simulink model "PMSM_FOC_Traction"  (R2020b)
settings: Solver=FixedStepAuto  StartTime=0.0  StopTime=10  RelTol=1e-3
model workspace (MAT data in the model file):
  wc : Simulink.Parameter (value not decoded)
values from neighbouring files (symbols this model uses):
  Cosine_table = 1.0 0.99999529 0.99999058 0.99998587 0.99998116 0.99996704 0.99995291 0.99993885 0.99992472 0.99990118 0.99987763 0.99985409 0.9998306 0.99979764 0.99976468 0.99973178 0.99969882 0.99965644 0.99961412 0.99957174 0.99952942 0.99947762 0.99942589 0.99937415 0.99932235 0.9992612 0.99920005 0.99913889 0.99907768 0.99900717 0.99893659 0.99886602 0.99879545 0.99871546 0.99863547 0.99855554 0.99847555 0.    [Hall_HSMO_FOC_Data.sldd]    (also in Hall_SMO_FOC_Data.sldd)
  Flux = 0.0109    [G474_FOC_HSMO.sldd]    (also in Hall_HSMO_FOC_Data.sldd = 0.00529276
  MTPA_id_table = 0.22889 0.23462678 0.23770036 0.2381243 0.23591207 0.23107713 0.2236329 0.21359272 0.20096992 0.18577772 0.16802935 0.14773798 0.12491672 0.099578641 0.071736768 0.041404068 0.0085934745 -0.026682133 -0.064409919 -0.10457709 -0.14717092 -0.1921787 -0.2395878 -0.28938559 -0.34155953 -0.39609709 -0.45298585 -0.51221335 -0.57376724 -0.63763517 -0.70380485 -0.77226412 -0.84300071 -0.91600245 -0.991257    [Hall_HSMO_FOC_Data.sldd]    (also in Hall_SMO_FOC_Data.sldd)
  MTPA_iq_table = -1.0417 -0.16083497 0.71926296 1.5985928 2.4771533 3.3549435 4.2319627 5.1082091 5.9836826 6.8583813 7.732305 8.6054525 9.4778223 10.349415 11.220228 12.090261 12.959513 13.827983 14.69567 15.562573 16.428694 17.294027 18.158575 19.022335 19.885307 20.747492 21.608887 22.469492 23.329306 24.188328 25.046556 25.903992 26.760633 27.616482 28.471533 29.325788 30.179247 31.031908 31.883772 32.734837 3    [Hall_HSMO_FOC_Data.sldd]    (also in Hall_SMO_FOC_Data.sldd)
  MTPA_Te_Max = 800.0    [Hall_HSMO_FOC_Data.sldd]    (also in Hall_SMO_FOC_Data.sldd)
  MTPA_Te_Min = 0.0    [Hall_HSMO_FOC_Data.sldd]    (also in Hall_SMO_FOC_Data.sldd)
  Sine_table = 0.0 0.0015339879 0.0030679768 0.0046019657 0.0061359555 0.0076698866 0.0092038177 0.010737749 0.012271681 0.013805497 0.015339312 0.016873131 0.018406944 0.019940587 0.021474229 0.023007872 0.024541514 0.026074925 0.027608337 0.029141748 0.03067516 0.032208283 0.033741407 0.035274528 0.036807653 0.038340431 0.039873205 0.04140598 0.042938754 0.04447113 0.046003502 0.047535874 0.049068246 0.0506001    [Hall_HSMO_FOC_Data.sldd]    (also in Hall_SMO_FOC_Data.sldd)
undefined symbols (not defined in the file or in its folder): CL_Param, ctrlParamsPI, DiscIntNeverNeededParam, Flux_weak, FluxObsever, Hall_Parameter, HFI, inverter, Kiv, Kiw, Kpv, Kpw, magnitude, OPL_Param, pmsm, Resolver_Parameter, sigbuilder_block, SMO, SVPWM, Vdc
libraries: powerlib x29, fl_lib x18, simulink x7, nesl_utility x7, pid_lib x5, dspstat3 x4, eeGeneralControl x4, eeDiscretePi x2, powerlib_extras x1, ee_lib x1
(part 4 of 6)

== system PMSM_FOC_Traction/Motor_Control/Motor_Control_Funtion/Angle_Speed_100us/SMO/Delta_theta ==
  Est_theta : Inport
  Ealpha_est : Inport  Port=2
  Ebeta_est : Inport  Port=3
  Add : Sum
  Add1 : Sum
  Divide : Product  Inputs=*/
  Gain : Gain  Gain=-1
  Math Function : Math  Operator=magnitude^2  SaturateOnIntegerOverflow=on
  Math Function1 : Math  Operator=magnitude^2  SaturateOnIntegerOverflow=on
  Product : Product
  Product1 : Product
  Saturation : Saturate  UpperLimit=inf  LowerLimit=4.0
  Sine_Cosine : Subsystem  TreatAsAtomicUnit=on
      settings: RTWSystemCode=Nonreusable function  RTWFcnNameOpts=Use subsystem name
  Sqrt : Sqrt  SaturateOnIntegerOverflow=on
  delta_theta : Outport
  unit : Outport  Port=2
  wires:
  Est_theta/1 -> Sine_Cosine/1(P)
  Ealpha_est/1 -> Math Function/1, Product/2
  Sine_Cosine/1(Sin) -> Product1/1
  Ebeta_est/1 -> Math Function1/1, Product1/2
  Product/1 -> Add/1
  Product1/1 -> Add/2
  Add/1 -> Gain/1
  Math Function/1 -> Add1/1
  Math Function1/1 -> Add1/2
  Add1/1 -> Sqrt/1
  Sqrt/1 -> Saturation/1
  Gain/1 -> Divide/1
  Saturation/1 -> unit/1, Divide/2
  Divide/1 -> delta_theta/1
  Sine_Cosine/2(Cos) -> Product/1

== system PMSM_FOC_Traction/Motor_Control/Motor_Control_Funtion/Angle_Speed_100us/SMO/PLL_PI ==
  in : Inport
  Add : Sum
  Discrete-Time Integrator : DiscreteIntegrator  SampleTime=Ts  ICPrevOutput=DiscIntNeverNeededParam  ICPrevScaledInput=DiscIntNeverNeededParam
  Gain2 : Gain  Gain=kp
  Gain3 : Gain  Gain=ki
  Saturation : Saturate  UpperLimit=inf  LowerLimit=-inf
  Scope : Scope  NumInputPorts=3
  Out : Outport
  wires:
  Gain2/1 -> Scope/1, Add/1
  Gain3/1 -> Discrete-Time Integrator/1
  Discrete-Time Integrator/1 -> Scope/2, Add/2
  in/1 -> Gain3/1, Gain2/1
  Add/1 -> Saturation/1
  Saturation/1 -> Scope/3, Out/1

== system PMSM_FOC_Traction/Motor_Control/Motor_Control_Funtion/Angle_Speed_100us/SMO/SMO_Fuction ==
  Ialpha : Inport
  Ibeta : Inport  Port=2
  Valpha : Inport  Port=3
  Vbeta : Inport  Port=4
  Est_we : Inport  Port=5
  Constant : Constant  Value=A  OutDataTypeStr=single
  Constant1 : Constant  Value=B  OutDataTypeStr=single
  Constant2 : Constant  Value=C  OutDataTypeStr=single
  Constant3 : Constant  Value=k  OutDataTypeStr=single
  Constant4 : Constant  Value=m  OutDataTypeStr=single
  Constant5 : Constant  Value=tao  OutDataTypeStr=single
  Constant6 : Constant  Value=Ts  OutDataTypeStr=single
  Display : Display
  S-Function Builder : S-Function  InitFcn=try, set_param(gcb,'FunctionName','SMO_Function'), end  FunctionName=SMO_Function  SFunctionModules=SMO_Function_wrapper  SFunctionDeploymentMode=off  EnableBusSupport=off  mask(S-Function Builder){}
      mask help: Simulink:masks:SFunctionBuilder_MD
      mask init:
      | val = [[.9  0.75 0.75 1 1 .9 .9 1]',[1 1 0.75 0.75 .9 .9 1 .9]'];try , sys = get_param(gcb,'SfunBuilderFcnName');if isempty(sys), sys = get_param(gcb,'FunctionName'); end,catch, sys = get_param(gcb,'FunctionName'); end
      settings: CopyFcn=set_param(gcbh,'LinkStatus','none')  PreSaveFcn=try, set_param(gcb,'FunctionName','SMO_Function'), end  OpenFcn=sfunctionwizard(gcbh)
      mask Display: plot(val(:,1),val(:,2)),disp(sys), port_label('input',1,'Ialpha'), port_label('input',2,'Ibeta'), port_label('input',3,'Valpha'), port_label('input',4,'Vbeta'), port_label('input',5,'Est_we'), port_label('input',6,'A'), port_label('input',7,'B'), port_label('input',8,'C'), port_label('input',9,'k'), port_label('input',10,'m'), port_label('input',11,'tao'), port_label('input',12,'Ts'), port_label('output',1,'Est_Ialpha'), port_label('output',2,'Est_Ibeta'), port_label('output',3,'Est_Ealpha'), port_label('output',4,'Est_Ebeta'), port_label('output',5,'Zalpha'), port_label('output',6,'Zbeta')
  Est_Ialpha : Outport
  Est_Ibeta : Outport  Port=2
  Est_Ealpha : Outport  Port=3
  Est_Ebeta : Outport  Port=4
  Zalpha : Outport  Port=5
  Zbeta : Outport  Port=6
  wires:
  S-Function Builder/4 -> Est_Ebeta/1
  S-Function Builder/6 -> Zbeta/1
  S-Function Builder/2 -> Est_Ibeta/1
  S-Function Builder/5 -> Zalpha/1
  S-Function Builder/3 -> Est_Ealpha/1
  S-Function Builder/1 -> Est_Ialpha/1
  Ialpha/1 -> S-Function Builder/1
  Ibeta/1 -> S-Function Builder/2
  Valpha/1 -> S-Function Builder/3
  Vbeta/1 -> S-Function Builder/4
  Est_we/1 -> S-Function Builder/5
  Constant/1 -> S-Function Builder/6, Display/1
  Constant1/1 -> S-Function Builder/7
  Constant2/1 -> S-Function Builder/8
  Constant3/1 -> S-Function Builder/9
  Constant4/1 -> S-Function Builder/10
  Constant5/1 -> S-Function Builder/11
  Constant6/1 -> S-Function Builder/12

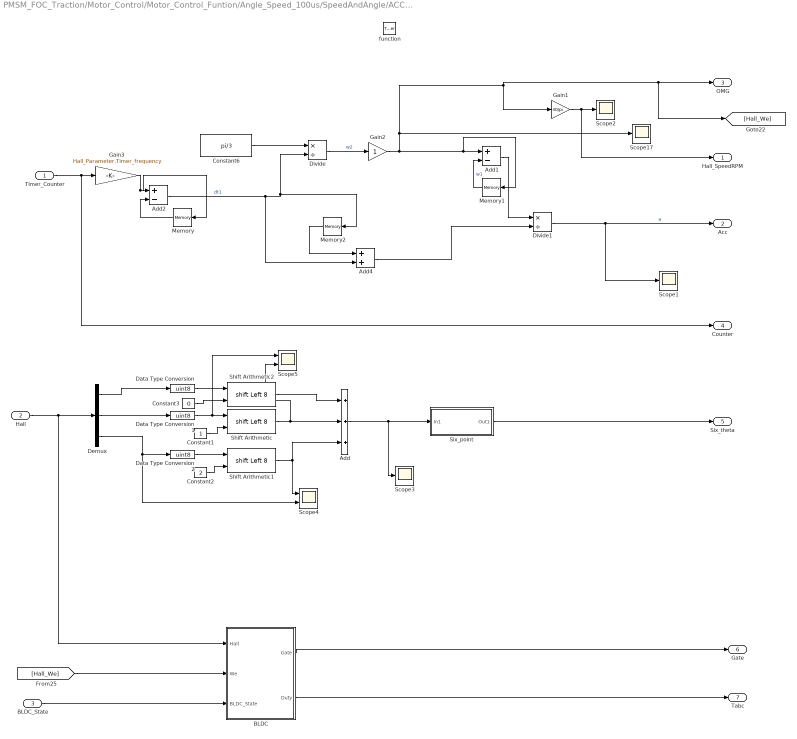
== system PMSM_FOC_Traction/Motor_Control/Motor_Control_Funtion/Angle_Speed_100us/SpeedAndAngle/ACC_OMG ==
  Timer_Counter : Inport
  Hall : Inport  Port=2
  BLDC_State : Inport  Port=3
  function : TriggerPort  TriggerType=either  VariantControl=Variant
  Add : Sum  Inputs=+++
  Add1 : Sum  Inputs=+-
  Add2 : Sum  Inputs=+-
  Add4 : Sum
  BLDC : Subsystem
  Constant1 : Constant  OutDataTypeStr=uint8
  Constant2 : Constant  Value=2  OutDataTypeStr=uint8
  Constant3 : Constant  Value=0  OutDataTypeStr=uint8
  Constant6 : Constant  Value=pi/3  OutDataTypeStr=single
  Data Type Conversion : DataTypeConversion  OutDataTypeStr=uint8
  Data Type Conversion1 : DataTypeConversion  OutDataTypeStr=uint8
  Data Type Conversion2 : DataTypeConversion  OutDataTypeStr=uint8
  Demux : Demux  Outputs=3
  Divide : Product  Inputs=*/
  Divide1 : Product  Inputs=*/
  Gain1 : Gain  Gain=30/pi  OutDataTypeStr=Inherit: Same as input  ParamDataTypeStr=Inherit: Same as input
  Gain2 : Gain  OutDataTypeStr=Inherit: Same as input  ParamDataTypeStr=Inherit: Same as input
  Gain3 : Gain  Gain=Hall_Parameter.Timer_frequency
  Memory : Memory  InheritSampleTime=on
  Memory1 : Memory  InheritSampleTime=on
  Memory2 : Memory  InheritSampleTime=on
  Scope{1..3,17} (4 alike) : Scope
  Scope4 : Scope  NumInputPorts=2
  Scope5 : Scope  NumInputPorts=2
  Shift Arithmetic : ArithShift  BitShiftNumberSource=Input port  BitShiftNumber=8  BitShiftDirection=Left
      settings: InputPortMap=u0,p1
  Shift Arithmetic1 : ArithShift  BitShiftNumberSource=Input port  BitShiftNumber=8  BitShiftDirection=Left
      settings: InputPortMap=u0,p1
  Shift Arithmetic2 : ArithShift  BitShiftNumberSource=Input port  BitShiftNumber=8  BitShiftDirection=Left
      settings: InputPortMap=u0,p1
  Six_point : Subsystem  TreatAsAtomicUnit=on
  Hall_SpeedRPM : Outport
  Acc : Outport  Port=2
  OMG : Outport  Port=3
  Counter : Outport  Port=4
  Six_theta : Outport  Port=5
  Gate : Outport  Port=6  VectorParamsAs1DForOutWhenUnconnected=off
  Tabc : Outport  Port=7  VectorParamsAs1DForOutWhenUnconnected=off
  wires:
  Timer_Counter/1 -> Counter/1, Gain3/1
  Constant6/1 -> Divide/1
  Divide/1 -> Gain2/1  "w2"
  Memory/1 -> Add2/2
  Add2/1 -> Add4/2, Memory2/1, Divide/2  "dt1"
  Memory1/1 -> Add1/2  "w1"
  Add1/1 -> Divide1/1
  Add4/1 -> Divide1/2
  Divide1/1 -> Acc/1, Scope1/1  "a"
  Gain3/1 -> Memory/1, Add2/1
  Gain1/1 -> Hall_SpeedRPM/1, Scope2/1
  Memory2/1 -> Add4/1
  Demux/3 -> Scope4/2, Data Type Conversion2/1
  Data Type Conversion2/1 -> Shift Arithmetic1/1
  Constant2/1 -> Shift Arithmetic1/2
  Constant1/1 -> Shift Arithmetic/2
  Data Type Conversion1/1 -> Scope5/1, Shift Arithmetic/1
  Demux/1 -> Data Type Conversion/1
  Shift Arithmetic/1 -> Add/2, Scope5/2
  Demux/2 -> Data Type Conversion1/1
  Six_point/1(Out1) -> Six_theta/1
  Gain2/1 -> Gain1/1, [Hall_We], OMG/1, Scope17/1, Memory1/1, Add1/1
  Shift Arithmetic1/1 -> Add/3, Scope4/1
  Add/1 -> Scope3/1, Six_point/1(In1)
  Data Type Conversion/1 -> Shift Arithmetic2/1
  Shift Arithmetic2/1 -> Add/1
  Constant3/1 -> Shift Arithmetic2/2
  Hall/1 -> BLDC/1(Hall), Demux/1
  [Hall_We] -> BLDC/2(We)
  BLDC/2(Duty) -> Tabc/1
  BLDC/1(Gate) -> Gate/1
  BLDC_State/1 -> BLDC/3(BLDC_State)

== system PMSM_FOC_Traction/Motor_Control/Motor_Control_Funtion/Angle_Speed_100us/SpeedAndAngle/ADC_IRQ ==
  Counter_ADC_IRQ : Inport
  Acc : Inport  Port=2
  OMG : Inport  Port=3
  Counter_Hall_IRQ : Inport  Port=4
  Six_theta : Inport  Port=5
  Add6 : Sum  Inputs=+-
  Add7 : Sum
  Gain2 : Gain  Gain=Hall_Parameter.Timer_frequency
  Gain3 : Gain  Gain=Hall_Parameter.Timer_frequency
  Gain4 : Gain  Gain=0.5
  Gain5 : Gain
  HallAngle_calibration : Subsystem
      settings: RTWSystemCode=Nonreusable function  RTWFcnNameOpts=Use subsystem name
  Math Function1 : Math  Operator=magnitude^2  SaturateOnIntegerOverflow=on
  Minus2 : Sum
  Product1 : Product
  Product2 : Product
  Hall_Angle : Outport
  wires:
  Gain5/1 -> Minus2/2
  Gain3/1 -> Math Function1/1
  Product2/1 -> Gain4/1
  Counter_Hall_IRQ/1 -> Add6/2
  Gain4/1 -> Minus2/1
  Add6/1 -> Gain3/1, Product1/2
  Math Function1/1 -> Product2/2
  Product1/1 -> Gain2/1
  Gain2/1 -> Gain5/1
  Counter_ADC_IRQ/1 -> Add6/1
  OMG/1 -> Product1/1
  Add7/1 -> HallAngle_calibration/1(Angle_input)
  Minus2/1 -> Add7/1
  Six_theta/1 -> Add7/2
  HallAngle_calibration/1(Angle_output) -> Hall_Angle/1  "SMO_Angle"
  Acc/1 -> Product2/1

== system PMSM_FOC_Traction/Motor_Control/Motor_Control_Funtion/Angle_Speed_100us/SpeedAndAngle/Subsystem ==
  BLDC_State : Inport
  Hall : Inport  Port=2
  If1 : If  IfExpression=u1 ==1  ElseIfExpressions=u1 ==2  ShowElse=off
  Merge : Merge
  Merge1 : Merge
  Subsystem : Subsystem
  Subsystem1 : Subsystem
  Gate : Outport  VectorParamsAs1DForOutWhenUnconnected=off
  Duty_Set : Outport  Port=2  VectorParamsAs1DForOutWhenUnconnected=off
  wires:
  BLDC_State/1 -> If1/1
  If1/1 -> Subsystem/Action
  If1/2 -> Subsystem1/Action
  Hall/1 -> Subsystem1/1(Hall)
  Subsystem/1(Gate) -> Merge/1
  Subsystem1/1(Gate) -> Merge/2
  Merge/1 -> Gate/1
  Subsystem/2(Duty_Set) -> Merge1/1
  Subsystem1/2(Duty_Set) -> Merge1/2
  Merge1/1 -> Duty_Set/1

== system PMSM_FOC_Traction/Motor_Control/Motor_Control_Funtion/Angle_Speed_100us/SpeedAndAngle/Subsystem1 ==
  Lock_Gate : Inport
  Lock_Duty : Inport  Port=2
  Hall_Gate : Inport  Port=3
  Hall_Duty : Inport  Port=4
  BLDC_State : Inport  Port=5
  If1 : If  IfExpression=u1 ==1 | u1 ==2  ElseIfExpressions=u1==3  ShowElse=off
  Merge : Merge
  Merge1 : Merge
  Subsystem : Subsystem
  Subsystem1 : Subsystem
  Gate : Outport  VectorParamsAs1DForOutWhenUnconnected=off
  Tabc : Outport  Port=2  VectorParamsAs1DForOutWhenUnconnected=off
  wires:
  BLDC_State/1 -> If1/1
  If1/1 -> Subsystem/Action
  Lock_Gate/1 -> Subsystem/1(In1)
  Lock_Duty/1 -> Subsystem/2(In2)
  If1/2 -> Subsystem1/Action
  Hall_Gate/1 -> Subsystem1/1(In1)
  Hall_Duty/1 -> Subsystem1/2(In2)
  Subsystem/1(Out1) -> Merge/1
  Subsystem1/1(Out1) -> Merge/2
  Merge/1 -> Gate/1
  Merge1/1 -> Tabc/1
  Subsystem/2(Out2) -> Merge1/1
  Subsystem1/2(Out2) -> Merge1/2

== system PMSM_FOC_Traction/Motor_Control/Motor_Control_Funtion/Angle_Speed_100us/Speed_Angle_Selector/Hall ==
  In1 : Inport
  In2 : Inport  Port=2
  Action Port : ActionPort  ActionPortLabel=if(u1==1)
  Out1 : Outport
  Out2 : Outport  Port=2
  wires:
  In1/1 -> Out1/1
  In2/1 -> Out2/1

== system PMSM_FOC_Traction/Motor_Control/Motor_Control_Funtion/Angle_Speed_100us/Speed_Angle_Selector/Resolver_Dir ==
  In1 : Inport
  In2 : Inport  Port=2
  Action Port : ActionPort  ActionPortLabel=if(u1==1)
  Out1 : Outport
  Out2 : Outport  Port=2
  wires:
  In1/1 -> Out1/1
  In2/1 -> Out2/1

== system PMSM_FOC_Traction/Motor_Control/Motor_Control_Funtion/Angle_Speed_100us/Speed_Angle_Selector/Resolver_PLL ==
  In1 : Inport
  In2 : Inport  Port=2
  Action Port : ActionPort  ActionPortLabel=if(u1==1)
  Out1 : Outport
  Out2 : Outport  Port=2
  wires:
  In1/1 -> Out1/1
  In2/1 -> Out2/1

== system PMSM_FOC_Traction/Motor_Control/Motor_Control_Funtion/Angle_Speed_100us/Speed_Angle_Selector/Sensorless ==
  In1 : Inport
  In2 : Inport  Port=2
  Action Port : ActionPort  ActionPortLabel=if(u1==1 | u2==1)
  Out1 : Outport
  Out2 : Outport  Port=2
  wires:
  In1/1 -> Out1/1
  In2/1 -> Out2/1

== system PMSM_FOC_Traction/Motor_Control/Motor_Control_Funtion/Angle_Speed_100us/Speed_Resolver/Speed_cacl ==
  position : Inport  OutMin=-4*pi  OutMax=4*pi
      settings: AttributesFormatString="------------------\\nMin =  %<OutMin>\\nMax =  %<OutMax>"
  Convert_to_Uint32 : DataTypeConversion  OutDataTypeStr=int32  RndMeth=Simplest
  Difference_Wrap : Sum  Inputs=+-  AccumDataTypeStr=int32  OutDataTypeStr=int32
  Difference_to_Single : DataTypeConversion  OutDataTypeStr=single
  LPF : DiscreteFilter  Numerator=[0 0.5]  Denominator=[1 -0.5]
  Position_Delay : Delay  DelayLength=1
  RPM_Gain : Gain  Gain=60/(2*pi*pmsm.PolePairs)  ParamDataTypeStr=single  OutDataTypeStr=single
      settings: AttributesFormatString=---------------------------------\n%<Gain>
  Scale_Input : Gain  Gain=((2^31) - 1)/(4*pi)  ParamDataTypeStr=single  OutDataTypeStr=single
      settings: AttributesFormatString=---------------------------------\n%<Gain>
  Scale_Output : Gain  Gain=pi/(2^31 -1)/(inverter.Ts)  ParamDataTypeStr=single  OutDataTypeStr=single
      settings: AttributesFormatString=---------------------------------\n%<Gain>
  Scope1 : Scope  NumInputPorts=2
  Scope7 : Scope  NumInputPorts=2
  Wrap_To_Pi : Gain  Gain=4  RndMeth=Simplest  OutDataTypeStr=Inherit: Same as input  ParamDataTypeStr=Inherit: Same as input
  Speed_RPM : Outport  VectorParamsAs1DForOutWhenUnconnected=off
  wires:
  position/1 -> Scale_Input/1  "position"
  Scale_Input/1 -> Convert_to_Uint32/1
  Difference_to_Single/1 -> Scope7/1, Scale_Output/1
  Wrap_To_Pi/1 -> Difference_Wrap/1, Position_Delay/1
  Scale_Output/1 -> RPM_Gain/1  "We"
  Position_Delay/1 -> Difference_Wrap/2
  Convert_to_Uint32/1 -> Wrap_To_Pi/1
  Difference_Wrap/1 -> Difference_to_Single/1
  RPM_Gain/1 -> Scope7/2, Scope1/2, LPF/1  "Speed_RPM"
  LPF/1 -> Scope1/1, Speed_RPM/1  "Speed_RPM_Filtered"

== system PMSM_FOC_Traction/Motor_Control/Motor_Control_Funtion/Angle_Speed_100us/Startup_OPL/Subsystem ==
  OPL_Speed : Inport
  OPL_Torque : Inport  Port=2
  Smo_theta : Inport  Port=3
  Action Port : ActionPort  ActionPortLabel=if(u1==2)
  2pi2 : Constant  Value=2*pi  OutDataTypeStr=single
  Constant1 : Constant  Value=1/OPL_Param.Acc_Times
  DT1 : DataTypeConversion  OutDataTypeStr=single
  DT2 : DataTypeConversion  OutDataTypeStr=single
  Discrete-Time Integrator1 : DiscreteIntegrator  SampleTime=-1  ICPrevOutput=DiscIntNeverNeededParam  ICPrevScaledInput=DiscIntNeverNeededParam
  Discrete-Time Integrator2 : DiscreteIntegrator  SampleTime=-1  ICPrevOutput=DiscIntNeverNeededParam  ICPrevScaledInput=DiscIntNeverNeededParam
  Mod2 : Math  Operator=mod  SaturateOnIntegerOverflow=on
  Product : Product
  Scope : Scope
  Scope1 : Scope
  Scope2 : Scope
  Scope3 : Scope  NumInputPorts=2
  Subtract : Sum  Inputs=+-
  We : Gain  Gain=pmsm.PolePairs*2*pi/60  OutDataTypeStr=single  ParamDataTypeStr=Inherit: Same as input
  Force_Angle : Outport
  OPL_Torque_Com : Outport  Port=2
  Delta_theta : Outport  Port=3
  Force_Switch : Outport  Port=4
  wires:
  DT1/1 -> Force_Angle/1  "Force_Angle"
  OPL_Torque/1 -> DT2/1
  DT2/1 -> OPL_Torque_Com/1
  We/1 -> Discrete-Time Integrator1/1  "Delta_Theta"
  2pi2/1 -> Mod2/2
  Mod2/1 -> Scope1/1, DT1/1  "Theta"
  OPL_Speed/1 -> Product/1
  Constant1/1 -> Product/2
  Product/1 -> Discrete-Time Integrator2/1
  Discrete-Time Integrator2/1 -> Scope/1, We/1
  Smo_theta/1 -> Scope3/1, Subtract/1
  Subtract/1 -> Scope2/1, Delta_theta/1
  Discrete-Time Integrator1/1 -> Scope3/2, Subtract/2, Force_Switch/1, Mod2/1

== system PMSM_FOC_Traction/Motor_Control/Motor_Control_Funtion/Angle_Speed_100us/Startup_OPL/Subsystem1 ==
  OPL_Torque : Inport
  Delta_theta : Inport  Port=2
  Force_RPM : Inport  Port=3
  Force_Switch : Inport  Port=4
  Action Port : ActionPort  ActionPortLabel=elseif(u1==3)
  2pi2 : Constant  Value=2*pi  OutDataTypeStr=single
  Constant1 : Constant  Value=1/OPL_Param.Revup_Times
  Constant2 : Constant  Value=1/OPL_Param.Revup_Times
  DT1 : DataTypeConversion  OutDataTypeStr=single
  DT2 : DataTypeConversion  OutDataTypeStr=single
  Discrete-Time Integrator1 : DiscreteIntegrator  SampleTime=-1  ICPrevOutput=DiscIntNeverNeededParam  ICPrevScaledInput=DiscIntNeverNeededParam
  Discrete-Time Integrator2 : DiscreteIntegrator  SampleTime=-1  ICPrevOutput=DiscIntNeverNeededParam  ICPrevScaledInput=DiscIntNeverNeededParam
  Discrete-Time Integrator3 : DiscreteIntegrator  SampleTime=-1  ICPrevOutput=DiscIntNeverNeededParam  ICPrevScaledInput=DiscIntNeverNeededParam
  Divide : Product  Inputs=*/
  Divide1 : Product  Inputs=*/
  Iq_Command : Constant  Value=OPL_Param.Current_ref/2  SampleTime=-1
  Mod2 : Math  Operator=mod  SaturateOnIntegerOverflow=on
  Subtract : Sum  Inputs=+++
  Subtract1 : Sum  Inputs=+-
  We : Gain  Gain=pmsm.PolePairs*2*pi/60  OutDataTypeStr=single  ParamDataTypeStr=Inherit: Same as input
  Force_Angle : Outport
  OPL_Torque_Com : Outport  Port=2
  Force_Angle1 : Outport  Port=3
  wires:
  DT2/1 -> OPL_Torque_Com/1
  Delta_theta/1 -> Divide/1
  Constant1/1 -> Divide/2
  Divide/1 -> Discrete-Time Integrator1/1
  Discrete-Time Integrator1/1 -> Subtract/1
  Force_RPM/1 -> We/1
  We/1 -> Discrete-Time Integrator2/1  "Delta_Theta"
  Force_Switch/1 -> Subtract/2
  Discrete-Time Integrator2/1 -> Subtract/3
  DT1/1 -> Force_Angle/1
  Subtract/1 -> Force_Angle1/1, Mod2/1
  Mod2/1 -> DT1/1  "Theta"
  2pi2/1 -> Mod2/2
  OPL_Torque/1 -> Subtract1/1
  Constant2/1 -> Divide1/2
  Iq_Command/1 -> Divide1/1
  Divide1/1 -> Discrete-Time Integrator3/1
  Discrete-Time Integrator3/1 -> Subtract1/2
  Subtract1/1 -> DT2/1

== system PMSM_FOC_Traction/Motor_Control/Motor_Control_Funtion/Control_Command_2ms/Speed_PI/Speed_PI ==
  PI_input : Inport
  HFI_State : Inport  Port=2
  Motor_State : Inport  Port=3
  Action Port : ActionPort  ActionPortLabel=if((u1==1)&(u2==3)|(u1~=1))
  HFI_Enalble : Constant  Value=HFI.Func_Enable  OutDataTypeStr=uint8
  If1 : If  NumInputs=3  IfExpression=(u1==3)&(u2==1)  ElseIfExpressions=(u2==0) & ((u3~=2)&(u3~=3))  ShowElse=off
  Merge : Merge
  Speed_Control : Subsystem
  Speed_Control1 : Subsystem
  PI_out : Outport  VectorParamsAs1DForOutWhenUnconnected=off
  wires:
  PI_input/1 -> Speed_Control1/1(Err), Speed_Control/1(Err)
  HFI_State/1 -> If1/1
  If1/1 -> Speed_Control/Action
  HFI_Enalble/1 -> If1/2
  If1/2 -> Speed_Control1/Action
  Merge/1 -> PI_out/1
  Speed_Control/1(PI_Out) -> Merge/1
  Speed_Control1/1(PI_Out) -> Merge/2
  Motor_State/1 -> If1/3

== system PMSM_FOC_Traction/Motor_Control/Motor_Control_Funtion/FOC_Control_100us/FOC/Angle_set ==
  Reso_angle : Inport
  HFI_angle : Inport  Port=2
  HFI_state : Inport  Port=3
  IPD_Angle : Inport  Port=4
  HFI_AngleEnable : Constant  Value=HFI.Angle_Enable  OutDataTypeStr=uint8
  If1 : If  IfExpression=u1 ==1
  Subsystem : Subsystem
  Subsystem1 : Subsystem
  Out1 : Outport
  Out2 : Outport  Port=2
  wires:
  HFI_AngleEnable/1 -> If1/1
  If1/1 -> Subsystem/Action
  HFI_angle/1 -> Subsystem/2(HFI_angle)
  If1/2 -> Subsystem1/Action
  Reso_angle/1 -> Subsystem1/1(Reso_angle)
  Subsystem/1(Out1) -> Out1/1
  Subsystem1/1(Out1) -> Out2/1
  HFI_state/1 -> Subsystem/1(HFI_state)
  IPD_Angle/1 -> Subsystem/3(IPD_Angle)

== system PMSM_FOC_Traction/Motor_Control/Motor_Control_Funtion/FOC_Control_100us/FOC/Clarke_Transform ==
  Phase_CurrentABC : Inport  PortDimensions=3
  Clark1 : Subsystem  TreatAsAtomicUnit=on
  Scope : Scope  NumInputPorts=2
  IAlpha : Outport  VectorParamsAs1DForOutWhenUnconnected=off
  IBeta : Outport  Port=2  VectorParamsAs1DForOutWhenUnconnected=off
  wires:
  Clark1/1(Ialpha) -> IAlpha/1, Scope/1
  Clark1/2(Ibeta) -> IBeta/1, Scope/2
  Phase_CurrentABC/1 -> Clark1/1(Iabc)

== system PMSM_FOC_Traction/Motor_Control/Motor_Control_Funtion/FOC_Control_100us/FOC/D_Current_PI ==
  Current_Command : Inport
  Current_Measured : Inport  Port=2
  Add2 : Sum  Inputs=|+-
  ID_Control : Subsystem
  Vd_voltage : Outport  VectorParamsAs1DForOutWhenUnconnected=off
  wires:
  Current_Command/1 -> Add2/1
  Current_Measured/1 -> Add2/2
  Add2/1 -> ID_Control/1(Err)  "currentControlError"
  ID_Control/1(PI_Out) -> Vd_voltage/1

== system PMSM_FOC_Traction/Motor_Control/Motor_Control_Funtion/FOC_Control_100us/FOC/Flux_weakening  ==
  Enable : Inport
  Vd : Inport  Port=2
  Vq : Inport  Port=3
  Id : Inport  Port=4
  Iq : Inport  Port=5
  If1 : If  IfExpression=u1 ==1
  Merge : Merge
  Merge1 : Merge
  Subsystem : Subsystem
  Subsystem1 : Subsystem
  Id_ref : Outport
  Iq_ref : Outport  Port=2
  wires:
  Enable/1 -> If1/1
  If1/1 -> Subsystem/Action
  If1/2 -> Subsystem1/Action
  Id/1 -> Subsystem/3(Id), Subsystem1/1(Id)
  Iq/1 -> Subsystem/4(Iq), Subsystem1/2(Iq)
  Vd/1 -> Subsystem/1(Vd)
  Vq/1 -> Subsystem/2(Vq)
  Subsystem/1(Id_ref) -> Merge/1
  Subsystem1/1(Id_ref) -> Merge/2
  Subsystem/2(Iq_ref) -> Merge1/1
  Subsystem1/2(Iq_ref) -> Merge1/2
  Merge1/1 -> Iq_ref/1
  Merge/1 -> Id_ref/1

== system PMSM_FOC_Traction/Motor_Control/Motor_Control_Funtion/FOC_Control_100us/FOC/HF_Observer ==
  Ialpha-beta : Inport
  Phase_CurrentABC : Inport  Port=2  PortDimensions=3
  Id : Inport  Port=3
  HFI_Enalble : Constant  Value=HFI.Func_Enable  OutDataTypeStr=uint8
  HFI_Function : Subsystem
      settings: RTWSystemCode=Nonreusable function  RTWFcnNameOpts=Use subsystem name
  If1 : If  IfExpression=u1==1  ShowElse=off
  RUN_State : Outport
  HFI_State : Outport  Port=2
  HFI_signal : Outport  Port=3
  speed_est : Outport  Port=4
  theta_est : Outport  Port=5
  Ualpha : Outport  Port=6
  Ubeta : Outport  Port=7
  IPD_Theta : Outport  Port=8
  wires:
  HFI_Function/1(RUN_State) -> RUN_State/1
  HFI_Function/3(HFI_signal) -> HFI_signal/1
  HFI_Function/4(speed_est) -> speed_est/1
  HFI_Function/5(theta_est) -> theta_est/1
  HFI_Function/7(Ubeta) -> Ubeta/1
  HFI_Function/6(Ualpha) -> Ualpha/1
  Id/1 -> HFI_Function/3(Id)
  Phase_CurrentABC/1 -> HFI_Function/2(Phase_CurrentABC)  "Phase_CurrentABC"
  Ialpha-beta/1 -> HFI_Function/1(Ialpha-beta)
  HFI_Enalble/1 -> If1/1
  If1/1 -> HFI_Function/Action
  HFI_Function/2(HFI_State) -> HFI_State/1
  HFI_Function/8(IPD_Theta) -> IPD_Theta/1

== system PMSM_FOC_Traction/Motor_Control/Motor_Control_Funtion/FOC_Control_100us/FOC/Inverse_Park_Transform ==
  D : Inport
  Q : Inport  Port=2
  Sin_Coefficient : Inport  Port=3
  Cos_Coefficient : Inport  Port=4
  Add1 : Sum  Inputs=+-  OutDataTypeStr=Inherit: Same as first input
  Add2 : Sum  OutDataTypeStr=Inherit: Same as first input
  Cos_Coefficient1 : InportShadow  Port=4
  Product{1..4} (4 alike) : Product  RndMeth=Simplest  OutDataTypeStr=Inherit: Same as first input
  Sin_Coefficient1 : InportShadow  Port=3
  Alpha : Outport  VectorParamsAs1DForOutWhenUnconnected=off
  Beta : Outport  Port=2  VectorParamsAs1DForOutWhenUnconnected=off
  wires:
  Add2/1 -> Beta/1
  Add1/1 -> Alpha/1
  Product3/1 -> Add2/1
  Product4/1 -> Add2/2
  Product1/1 -> Add1/1
  Product2/1 -> Add1/2
  Cos_Coefficient1/1 -> Product4/2
  Sin_Coefficient/1 -> Product2/2
  D/1 -> Product3/1, Product1/1
  Q/1 -> Product2/1, Product4/1
  Sin_Coefficient1/1 -> Product3/2
  Cos_Coefficient/1 -> Product1/2

== system PMSM_FOC_Traction/Motor_Control/Motor_Control_Funtion/FOC_Control_100us/FOC/Park_Transform ==
  Alpha : Inport
  Beta : Inport  Port=2
  Sin_Coefficient : Inport  Port=3
  Cos_Coefficient : Inport  Port=4
  Add1 : Sum  OutDataTypeStr=Inherit: Same as first input
  Add2 : Sum  Inputs=-+  OutDataTypeStr=Inherit: Same as first input
  Alpha1 : InportShadow
  Beta1 : InportShadow  Port=2
  Cos_Coefficient1 : InportShadow  Port=4
  Produc3t : Product  RndMeth=Simplest  OutDataTypeStr=Inherit: Same as first input
  Product1 : Product  RndMeth=Simplest  OutDataTypeStr=Inherit: Same as first input
  Product2 : Product  RndMeth=Simplest  OutDataTypeStr=Inherit: Same as first input
  Product4 : Product  RndMeth=Simplest  OutDataTypeStr=Inherit: Same as first input
  Sin_Coefficient1 : InportShadow  Port=3
  D : Outport  VectorParamsAs1DForOutWhenUnconnected=off
  Q : Outport  Port=2  VectorParamsAs1DForOutWhenUnconnected=off
  wires:
  Produc3t/1 -> Add2/1
  Product4/1 -> Add2/2
  Product1/1 -> Add1/1
  Product2/1 -> Add1/2
  Alpha1/1 -> Produc3t/1
  Sin_Coefficient1/1 -> Produc3t/2
  Cos_Coefficient1/1 -> Product4/2
  Beta1/1 -> Product4/1
  Alpha/1 -> Product1/1
  Cos_Coefficient/1 -> Product1/2
  Beta/1 -> Product2/1
  Sin_Coefficient/1 -> Product2/2
  Add1/1 -> D/1
  Add2/1 -> Q/1

== system PMSM_FOC_Traction/Motor_Control/Motor_Control_Funtion/FOC_Control_100us/FOC/Q_Current_PI ==
  Current_Command : Inport
  Current_Measured : Inport  Port=2
  Add2 : Sum  Inputs=|+-
  IQ_Control : Subsystem
  Vq_voltage : Outport  VectorParamsAs1DForOutWhenUnconnected=off
  wires:
  Current_Command/1 -> Add2/1
  Current_Measured/1 -> Add2/2
  Add2/1 -> IQ_Control/1(Err)  "currentControlError"
  IQ_Control/1(PI_Out) -> Vq_voltage/1

== system PMSM_FOC_Traction/Motor_Control/Motor_Control_Funtion/FOC_Control_100us/FOC/SVPWM ==
  Valpha : Inport
  Vbeta : Inport  Port=2
  Vdc : Inport  Port=3
  Ts : Inport  Port=4
  Gain : Gain  Gain=83990000
  Gain2 : Gain  Gain=83990000
  Gain3 : Gain  Gain=83990000
  N Sector  Caculate : Subsystem  TreatAsAtomicUnit=on
  T1 T2  Caculate : Subsystem  TreatAsAtomicUnit=on
  Tcm calculate : Subsystem  TreatAsAtomicUnit=on
  XYZ Caculate : Subsystem  TreatAsAtomicUnit=on
  Ta : Outport
  Tb : Outport  Port=2
  Tc : Outport  Port=3
  wires:
  Tcm calculate/2(Tcm2) -> Gain2/1
  Tcm calculate/3(Tcm3) -> Gain3/1
  Tcm calculate/1(Tcm1) -> Gain/1
  T1 T2  Caculate/2(T2) -> Tcm calculate/3(T2)
  XYZ Caculate/1(X) -> T1 T2  Caculate/2(X)
  N Sector  Caculate/1(N) -> T1 T2  Caculate/1(N), Tcm calculate/1(N)
  Vdc/1 -> XYZ Caculate/3(Udc)
  T1 T2  Caculate/1(T1) -> Tcm calculate/2(T1)
  XYZ Caculate/3(Z) -> T1 T2  Caculate/4(Z)
  XYZ Caculate/2(Y) -> T1 T2  Caculate/3(Y)
  Valpha/1 -> N Sector  Caculate/2(Ualf), XYZ Caculate/1(Ualfpa)
  Vbeta/1 -> N Sector  Caculate/1(Ubelta), XYZ Caculate/2(Ubelta)
  Ts/1 -> T1 T2  Caculate/5(Tpwm), Tcm calculate/4(Tpwm), XYZ Caculate/4(Tpwm)
  Gain/1 -> Ta/1
  Gain3/1 -> Tc/1
  Gain2/1 -> Tb/1

== system PMSM_FOC_Traction/Motor_Control/Motor_Control_Funtion/FOC_Control_100us/FOC/Set_Idq ==
  HFI_state : Inport
  Id_Command : Inport  Port=2
  Iq_Command : Inport  Port=3
  Constant1 : Constant  Value=0  OutDataTypeStr=single
  Constant2 : Constant  Value=0  OutDataTypeStr=single
  If1 : If  IfExpression=u1==2 | u1==1
  Merge : Merge
  Merge1 : Merge
  Set_Idq : Subsystem  TreatAsAtomicUnit=on
      settings: RTWSystemCode=Nonreusable function  RTWFcnNameOpts=Use subsystem name
  Set_Idq1 : Subsystem  TreatAsAtomicUnit=on
      settings: RTWSystemCode=Nonreusable function  RTWFcnNameOpts=Use subsystem name
  Id : Outport  VectorParamsAs1DForOutWhenUnconnected=off
  Iq : Outport  Port=2  VectorParamsAs1DForOutWhenUnconnected=off
  wires:
  HFI_state/1 -> If1/1
  Constant2/1 -> Set_Idq/1(Id_Command)
  Constant1/1 -> Set_Idq/2(Iq_Command)
  Id_Command/1 -> Set_Idq1/1(Id_Command)
  Iq_Command/1 -> Set_Idq1/2(Iq_Command)
  If1/1 -> Set_Idq/Action
  If1/2 -> Set_Idq1/Action
  Set_Idq/1(Id) -> Merge/1
  Set_Idq1/1(Id) -> Merge/2
  Merge/1 -> Id/1
  Set_Idq/2(Iq) -> Merge1/1
  Set_Idq1/2(Iq) -> Merge1/2
  Merge1/1 -> Iq/1

== system PMSM_FOC_Traction/Motor_Control/Motor_Control_Funtion/FOC_Control_100us/FOC/Sine_Cosine ==
  note: Sine Cosine Coefficients
  P : Inport
  Cosine : Lookup_n-D  NumberOfTableDimensions=1  LookupTableObject=''  BreakpointsForDimension1=[0:2*pi/4095:2*pi]  BreakpointsForDimension1FirstPoint=10  BreakpointsForDimension2FirstPoint=10  BreakpointsForDimension1Spacing=12  BreakpointsForDimension2Spacing=12  IndexSearchMethod=Evenly spaced points  Table=Cosine_table  InterpMethod=Flat  DiagnosticForOutOfRangeInput=Error  InternalRulePriority=Speed  RndMeth=Simplest  InputSameDT=on
  Saturation : Saturate  UpperLimit=2*pi-0.0001  LowerLimit=0+0.0001
  Scope : Scope  NumInputPorts=2
  Sine : Lookup_n-D  NumberOfTableDimensions=1  LookupTableObject=''  BreakpointsForDimension1=[0:2*pi/4095:2*pi]  BreakpointsForDimension1FirstPoint=10  BreakpointsForDimension2FirstPoint=10  BreakpointsForDimension1Spacing=12  BreakpointsForDimension2Spacing=12  IndexSearchMethod=Evenly spaced points  Table=Sine_table  InterpMethod=Flat  DiagnosticForOutOfRangeInput=Error  InternalRulePriority=Speed  RndMeth=Simplest  InputSameDT=on
  Sin : Outport  VectorParamsAs1DForOutWhenUnconnected=off
  Cos : Outport  Port=2  VectorParamsAs1DForOutWhenUnconnected=off
  wires:
  P/1 -> Saturation/1  "position"
  Sine/1 -> Scope/1, Sin/1
  Cosine/1 -> Scope/2, Cos/1
  Saturation/1 -> Cosine/1, Sine/1

== system PMSM_FOC_Traction/Motor_Control/Motor_Control_Funtion/FOC_Control_100us/FOC/Subsystem1 ==
  HFI_State : Inport
  HFI_Ualpha : Inport  Port=2
  HFI_Ubeta : Inport  Port=3
  Ualpha : Inport  Port=4
  Ubeta : Inport  Port=5
  If Action Subsystem1 : Subsystem  TreatAsAtomicUnit=on
  If Action Subsystem2 : Subsystem  TreatAsAtomicUnit=on
  If1 : If  IfExpression=(u1<3)&(u1>0)
  Merge : Merge
  Merge1 : Merge
  Ualpha_out : Outport
  Ubeta_out : Outport  Port=2
  wires:
  If1/1 -> If Action Subsystem2/Action
  If1/2 -> If Action Subsystem1/Action
  HFI_Ualpha/1 -> If Action Subsystem2/1(In1)
  HFI_Ubeta/1 -> If Action Subsystem2/2(In2)
  Ualpha/1 -> If Action Subsystem1/1(In1)
  Ubeta/1 -> If Action Subsystem1/2(In2)
  If Action Subsystem2/1(Out1) -> Merge/1
  If Action Subsystem1/1(Out1) -> Merge/2
  If Action Subsystem2/2(Out2) -> Merge1/1
  If Action Subsystem1/2(Out2) -> Merge1/2
  Merge/1 -> Ualpha_out/1
  Merge1/1 -> Ubeta_out/1
  HFI_State/1 -> If1/1

== system PMSM_FOC_Traction/Motor_Control/Motor_Control_Funtion/FOC_Control_100us/Iq_selector/Subsystem ==
  In1 : Inport
  Action Port : ActionPort  ActionPortLabel=if(u1 ==2 | u1 ==3)
  Out1 : Outport
  wires:
  In1/1 -> Out1/1

== system PMSM_FOC_Traction/Motor_Control/Motor_Control_Funtion/FOC_Control_100us/Iq_selector/Subsystem1 ==
  In1 : Inport
  Action Port : ActionPort  ActionPortLabel=else
  Out1 : Outport
  wires:
  In1/1 -> Out1/1

== system PMSM_FOC_Traction/PMSM/Control/Control/Commutation/Bit concatenate ==
  u : Inport
  Gain : Gain  Gain=[4 2 1]  Multiplication=Matrix(K*u)
  Sum of Elements : Sum  Inputs=+
  y : Outport  VectorParamsAs1DForOutWhenUnconnected=off
  wires:
  u/1 -> Gain/1
  Gain/1 -> Sum of Elements/1
  Sum of Elements/1 -> y/1

== system PMSM_FOC_Traction/PMSM/SpeedAndAngle/ACC_OMG/Six_point/Sector_1 ==
  Action Port : ActionPort  ActionPortLabel=case [ 1 ]:
  Add : Sum
  Constant : Constant  Value=Hall_Parameter.Sector_1  OutDataTypeStr=single
  Constant1 : Constant  Value=Hall_Parameter.shift  OutDataTypeStr=single
  Angle_0 : Outport
  wires:
  Constant/1 -> Add/1
  Constant1/1 -> Add/2
  Add/1 -> Angle_0/1

== system PMSM_FOC_Traction/PMSM/SpeedAndAngle/ACC_OMG/Six_point/Sector_2 ==
  Action Port : ActionPort  ActionPortLabel=case [ 2 ]:
  Add : Sum
  Constant1 : Constant  Value=Hall_Parameter.shift  OutDataTypeStr=single
  Pi/3 : Constant  Value=Hall_Parameter.Sector_2  OutDataTypeStr=single
  Angle_0 : Outport
  wires:
  Pi/3/1 -> Add/1
  Constant1/1 -> Add/2
  Add/1 -> Angle_0/1

== system PMSM_FOC_Traction/PMSM/SpeedAndAngle/ACC_OMG/Six_point/Sector_3 ==
  Action Port : ActionPort  ActionPortLabel=case [ 3 ]:
  Add : Sum
  Constant : Constant  Value=Hall_Parameter.Sector_3  OutDataTypeStr=single
  Constant1 : Constant  Value=Hall_Parameter.shift  OutDataTypeStr=single
  Angle_0 : Outport
  wires:
  Constant/1 -> Add/1
  Add/1 -> Angle_0/1
  Constant1/1 -> Add/2

== system PMSM_FOC_Traction/PMSM/SpeedAndAngle/ACC_OMG/Six_point/Sector_4 ==
  Action Port : ActionPort  ActionPortLabel=case [ 4 ]:
  Add : Sum
  Constant : Constant  Value=Hall_Parameter.Sector_4  OutDataTypeStr=single
  Constant1 : Constant  Value=Hall_Parameter.shift  OutDataTypeStr=single
  Angle_0 : Outport
  wires:
  Constant/1 -> Add/1
  Add/1 -> Angle_0/1
  Constant1/1 -> Add/2

== system PMSM_FOC_Traction/PMSM/SpeedAndAngle/ACC_OMG/Six_point/Sector_5 ==
  Action Port : ActionPort  ActionPortLabel=case [ 5 ]:
  Add : Sum
  Constant : Constant  Value=Hall_Parameter.Sector_5  OutDataTypeStr=single
  Constant1 : Constant  Value=Hall_Parameter.shift  OutDataTypeStr=single
  Angle_0 : Outport
  wires:
  Constant/1 -> Add/1
  Add/1 -> Angle_0/1
  Constant1/1 -> Add/2

== system PMSM_FOC_Traction/PMSM/SpeedAndAngle/ACC_OMG/Six_point/Sector_6 ==
  Action Port : ActionPort  ActionPortLabel=case [ 6 ]:
  Add : Sum
  Constant : Constant  Value=Hall_Parameter.Sector_6  OutDataTypeStr=single
  Constant1 : Constant  Value=Hall_Parameter.shift  OutDataTypeStr=single
  Angle_0 : Outport
  wires:
  Constant/1 -> Add/1
  Add/1 -> Angle_0/1
  Constant1/1 -> Add/2

== system PMSM_FOC_Traction/PMSM/SpeedAndAngle/ADC_IRQ/HallAngle_calibration/If Action Subsystem1 ==
  In1 : Inport
  Action Port : ActionPort  ActionPortLabel=else
  Out1 : Outport
  wires:
  In1/1 -> Out1/1

== system PMSM_FOC_Traction/PMSM/SpeedAndAngle/ADC_IRQ/HallAngle_calibration/If Action Subsystem2 ==
  In1 : Inport
  Action Port : ActionPort  ActionPortLabel=if(u1 > 6.283185307)
  2pi : Constant  Value=2*pi  OutDataTypeStr=single
  Subtract1 : Sum  Inputs=+-  OutDataTypeStr=single
  Out1 : Outport
  wires:
  In1/1 -> Subtract1/1
  Subtract1/1 -> Out1/1
  2pi/1 -> Subtract1/2

== system PMSM_FOC_Traction/PMSM/SpeedAndAngle/ADC_IRQ/HallAngle_calibration/If Action Subsystem3 ==
  In1 : Inport
  Action Port : ActionPort  ActionPortLabel=elseif(u1<0)
  Angle_offset : Constant  Value=2*pi  OutDataTypeStr=single
  Subtract1 : Sum
  Out1 : Outport
  wires:
  In1/1 -> Subtract1/1
  Subtract1/1 -> Out1/1
  Angle_offset/1 -> Subtract1/2

== system PMSM_FOC_Traction/Motor_Control/Motor_Control_Funtion/Angle_Speed_100us/Flux_OBSERVER/equ3.12/Sine_Cosine ==
  note: Sine Cosine Coefficients
  P : Inport
  Cosine : Lookup_n-D  NumberOfTableDimensions=1  LookupTableObject=''  BreakpointsForDimension1=[0:2*pi/4095:2*pi]  BreakpointsForDimension1FirstPoint=10  BreakpointsForDimension2FirstPoint=10  BreakpointsForDimension1Spacing=12  BreakpointsForDimension2Spacing=12  IndexSearchMethod=Evenly spaced points  Table=Cosine_table  InterpMethod=Flat  DiagnosticForOutOfRangeInput=Error  InternalRulePriority=Speed  RndMeth=Simplest  InputSameDT=on
  Saturation : Saturate  UpperLimit=2*pi-0.0001  LowerLimit=0+0.0001
  Scope : Scope  NumInputPorts=2
  Sine : Lookup_n-D  NumberOfTableDimensions=1  LookupTableObject=''  BreakpointsForDimension1=[0:2*pi/4095:2*pi]  BreakpointsForDimension1FirstPoint=10  BreakpointsForDimension2FirstPoint=10  BreakpointsForDimension1Spacing=12  BreakpointsForDimension2Spacing=12  IndexSearchMethod=Evenly spaced points  Table=Sine_table  InterpMethod=Flat  DiagnosticForOutOfRangeInput=Error  InternalRulePriority=Speed  RndMeth=Simplest  InputSameDT=on
  Sin : Outport  VectorParamsAs1DForOutWhenUnconnected=off
  Cos : Outport  Port=2  VectorParamsAs1DForOutWhenUnconnected=off
  wires:
  P/1 -> Saturation/1  "position"
  Sine/1 -> Scope/1, Sin/1
  Cosine/1 -> Scope/2, Cos/1
  Saturation/1 -> Cosine/1, Sine/1

== system PMSM_FOC_Traction/Motor_Control/Motor_Control_Funtion/Angle_Speed_100us/Flux_OBSERVER/equ3.12/integrator ==
  x(k) : Inport  OutDataTypeStr=single
  RangeLimit : Subsystem
  Sum1 : Sum  Inputs=|++  OutDataTypeStr=single
  Ts : Gain  Gain=inverter.Ts  OutDataTypeStr=single
  Unit Delay : UnitDelay  SampleTime=-1  HasFrameUpgradeWarning=on
  y(k-1) : Outport  OutDataTypeStr=single
  wires:
  x(k)/1 -> Ts/1
  Ts/1 -> Sum1/1
  Sum1/1 -> RangeLimit/1(In)  "y(k)"
  Unit Delay/1 -> y(k-1)/1, Sum1/2
  RangeLimit/1(Theta) -> Unit Delay/1

== system PMSM_FOC_Traction/Motor_Control/Motor_Control_Funtion/Angle_Speed_100us/HIGH_SMO/QPLL/SpeedToTheta ==
  In1 : Inport
  RangeLimit : Subsystem
  Sum1 : Sum  Inputs=|++
  Ts : Gain  Gain=inverter.Ts
  Unit Delay : UnitDelay  SampleTime=-1  HasFrameUpgradeWarning=on
  sin_cos : Outport
  wires:
  In1/1 -> Ts/1
  Ts/1 -> Sum1/1
  Sum1/1 -> RangeLimit/1(In)
  Unit Delay/1 -> sin_cos/1, Sum1/2
  RangeLimit/1(Theta) -> Unit Delay/1

== system PMSM_FOC_Traction/Motor_Control/Motor_Control_Funtion/Angle_Speed_100us/HIGH_SMO/QPLL/Subsystem1 ==
  Err_in : Inport
  speed : Inport  Port=2
  If : If
  If Action Subsystem : Subsystem  TreatAsAtomicUnit=on
  If Action Subsystem1 : Subsystem  TreatAsAtomicUnit=on
  Merge : Merge
  Product : Product
  Out : Outport  VectorParamsAs1DForOutWhenUnconnected=off
  wires:
  speed/1 -> If/1
  Merge/1 -> Product/1
  Err_in/1 -> Product/2
  Product/1 -> Out/1
  If/1 -> If Action Subsystem/Action
  If Action Subsystem/1(Out1) -> Merge/1
  If Action Subsystem1/1(Out1) -> Merge/2
  If/2 -> If Action Subsystem1/Action

== system PMSM_FOC_Traction/Motor_Control/Motor_Control_Funtion/Angle_Speed_100us/Resolver_Observer/Angle_calibration/If Action Subsystem1 ==
  In1 : Inport
  Action Port : ActionPort  ActionPortLabel=else
  Out1 : Outport
  wires:
  In1/1 -> Out1/1

== system PMSM_FOC_Traction/Motor_Control/Motor_Control_Funtion/Angle_Speed_100us/Resolver_Observer/Angle_calibration/If Action Subsystem2 ==
  In1 : Inport
  Action Port : ActionPort  ActionPortLabel=if(u1 > 6.283185307)
  2pi : Constant  Value=2*pi  OutDataTypeStr=single
  Subtract1 : Sum  Inputs=+-  OutDataTypeStr=single
  Out1 : Outport
  wires:
  In1/1 -> Subtract1/1
  Subtract1/1 -> Out1/1
  2pi/1 -> Subtract1/2

== system PMSM_FOC_Traction/Motor_Control/Motor_Control_Funtion/Angle_Speed_100us/Resolver_Observer/Angle_calibration/If Action Subsystem3 ==
  In1 : Inport
  Action Port : ActionPort  ActionPortLabel=elseif(u1<0)
  Angle_offset : Constant  Value=2*pi  OutDataTypeStr=single
  Subtract1 : Sum
  Out1 : Outport
  wires:
  In1/1 -> Subtract1/1
  Subtract1/1 -> Out1/1
  Angle_offset/1 -> Subtract1/2

== system PMSM_FOC_Traction/Motor_Control/Motor_Control_Funtion/Angle_Speed_100us/Resolver_Observer/Resolver_Angle_cacl/Sine_Cosine ==
  note: Sine Cosine Coefficients
  P : Inport
  Cosine : Lookup_n-D  NumberOfTableDimensions=1  LookupTableObject=''  BreakpointsForDimension1=[0:2*pi/4095:2*pi]  BreakpointsForDimension1FirstPoint=10  BreakpointsForDimension2FirstPoint=10  BreakpointsForDimension1Spacing=12  BreakpointsForDimension2Spacing=12  IndexSearchMethod=Evenly spaced points  Table=Cosine_table  InterpMethod=Flat  DiagnosticForOutOfRangeInput=Error  InternalRulePriority=Speed  RndMeth=Simplest  InputSameDT=on
  Saturation : Saturate  UpperLimit=2*pi-0.0001  LowerLimit=0+0.0001
  Scope : Scope  NumInputPorts=2
  Sine : Lookup_n-D  NumberOfTableDimensions=1  LookupTableObject=''  BreakpointsForDimension1=[0:2*pi/4095:2*pi]  BreakpointsForDimension1FirstPoint=10  BreakpointsForDimension2FirstPoint=10  BreakpointsForDimension1Spacing=12  BreakpointsForDimension2Spacing=12  IndexSearchMethod=Evenly spaced points  Table=Sine_table  InterpMethod=Flat  DiagnosticForOutOfRangeInput=Error  InternalRulePriority=Speed  RndMeth=Simplest  InputSameDT=on
  Sin : Outport  VectorParamsAs1DForOutWhenUnconnected=off
  Cos : Outport  Port=2  VectorParamsAs1DForOutWhenUnconnected=off
  wires:
  P/1 -> Saturation/1  "position"
  Sine/1 -> Scope/1, Sin/1
  Cosine/1 -> Scope/2, Cos/1
  Saturation/1 -> Cosine/1, Sine/1

== system PMSM_FOC_Traction/Motor_Control/Motor_Control_Funtion/Angle_Speed_100us/SMO/Angle_calibration/If Action Subsystem1 ==
  In1 : Inport
  Action Port : ActionPort  ActionPortLabel=else
  Out1 : Outport
  wires:
  In1/1 -> Out1/1

== system PMSM_FOC_Traction/Motor_Control/Motor_Control_Funtion/Angle_Speed_100us/SMO/Angle_calibration/If Action Subsystem2 ==
  In1 : Inport
  Action Port : ActionPort  ActionPortLabel=if(u1 > 6.283185307)
  2pi : Constant  Value=2*pi  OutDataTypeStr=single
  Subtract1 : Sum  Inputs=+-  OutDataTypeStr=single
  Out1 : Outport
  wires:
  In1/1 -> Subtract1/1
  Subtract1/1 -> Out1/1
  2pi/1 -> Subtract1/2

== system PMSM_FOC_Traction/Motor_Control/Motor_Control_Funtion/Angle_Speed_100us/SMO/Angle_calibration/If Action Subsystem3 ==
  In1 : Inport
  Action Port : ActionPort  ActionPortLabel=elseif(u1<0)
  Angle_offset : Constant  Value=2*pi  OutDataTypeStr=single
  Subtract1 : Sum
  Out1 : Outport
  wires:
  In1/1 -> Subtract1/1
  Subtract1/1 -> Out1/1
  Angle_offset/1 -> Subtract1/2

== system PMSM_FOC_Traction/Motor_Control/Motor_Control_Funtion/Angle_Speed_100us/SMO/Delta_theta/Sine_Cosine ==
  note: Sine Cosine Coefficients
  P : Inport
  Cosine : Lookup_n-D  NumberOfTableDimensions=1  LookupTableObject=''  BreakpointsForDimension1=[0:2*pi/4095:2*pi]  BreakpointsForDimension1FirstPoint=10  BreakpointsForDimension2FirstPoint=10  BreakpointsForDimension1Spacing=12  BreakpointsForDimension2Spacing=12  IndexSearchMethod=Evenly spaced points  Table=Cosine_table  InterpMethod=Flat  DiagnosticForOutOfRangeInput=Error  InternalRulePriority=Speed  RndMeth=Simplest  InputSameDT=on
  Saturation : Saturate  UpperLimit=2*pi-0.0001  LowerLimit=0+0.0001
  Scope : Scope  NumInputPorts=2
  Sine : Lookup_n-D  NumberOfTableDimensions=1  LookupTableObject=''  BreakpointsForDimension1=[0:2*pi/4095:2*pi]  BreakpointsForDimension1FirstPoint=10  BreakpointsForDimension2FirstPoint=10  BreakpointsForDimension1Spacing=12  BreakpointsForDimension2Spacing=12  IndexSearchMethod=Evenly spaced points  Table=Sine_table  InterpMethod=Flat  DiagnosticForOutOfRangeInput=Error  InternalRulePriority=Speed  RndMeth=Simplest  InputSameDT=on
  Sin : Outport  VectorParamsAs1DForOutWhenUnconnected=off
  Cos : Outport  Port=2  VectorParamsAs1DForOutWhenUnconnected=off
  wires:
  P/1 -> Saturation/1  "position"
  Sine/1 -> Scope/1, Sin/1
  Cosine/1 -> Scope/2, Cos/1
  Saturation/1 -> Cosine/1, Sine/1

== system PMSM_FOC_Traction/Motor_Control/Motor_Control_Funtion/Angle_Speed_100us/SpeedAndAngle/ACC_OMG/BLDC ==
  Hall : Inport
  We : Inport  Port=2
  BLDC_State : Inport  Port=3
  Control : Subsystem
  Low pass filter : DiscreteTransferFcn  Numerator=[1-exp(-2*pi*20*inverter.Ts)]  Denominator=[1 -exp(-2*pi*20*inverter.Ts)]
  Scope : Scope  NumInputPorts=2
  T3 : Constant  Value=1000  OutDataTypeStr=single
  Gate : Outport  VectorParamsAs1DForOutWhenUnconnected=off
  Duty : Outport  Port=2  VectorParamsAs1DForOutWhenUnconnected=off
  wires:
  Hall/1 -> Control/3(Hall)
  T3/1 -> Control/1(RPMReq)
  We/1 -> Scope/2, Low pass filter/1
  Control/1(Gate) -> Gate/1
  Control/2(Duty) -> Duty/1
  Low pass filter/1 -> Scope/1, Control/2(w_sens)
  BLDC_State/1 -> Control/4(BLDC_State)

== system PMSM_FOC_Traction/Motor_Control/Motor_Control_Funtion/Angle_Speed_100us/SpeedAndAngle/ACC_OMG/Six_point ==
  In1 : Inport
  Merge2 : Merge  Inputs=6
  Scope : Scope  NumInputPorts=2
  Sector_1 : Subsystem
  Sector_2 : Subsystem
  Sector_3 : Subsystem
  Sector_4 : Subsystem
  Sector_5 : Subsystem
  Sector_6 : Subsystem
  Switch Case2 : SwitchCase  CaseConditions={1,2,3,4,5,6}  ShowDefaultCase=off
  Out1 : Outport
  wires:
  Sector_4/1(Angle_0) -> Merge2/4
  Switch Case2/5 -> Sector_5/Action
  Sector_6/1(Angle_0) -> Merge2/6
  Sector_5/1(Angle_0) -> Merge2/5
  Switch Case2/6 -> Sector_6/Action
  Switch Case2/3 -> Sector_3/Action
  Switch Case2/4 -> Sector_4/Action
  Sector_1/1(Angle_0) -> Merge2/1
  Switch Case2/2 -> Sector_2/Action
  In1/1 -> Scope/1, Switch Case2/1
  Sector_3/1(Angle_0) -> Merge2/3
  Switch Case2/1 -> Sector_1/Action
  Sector_2/1(Angle_0) -> Merge2/2
  Merge2/1 -> Scope/2, Out1/1

== system PMSM_FOC_Traction/Motor_Control/Motor_Control_Funtion/Angle_Speed_100us/SpeedAndAngle/ADC_IRQ/HallAngle_calibration ==
  Angle_input : Inport
  Angle_offset : Constant  Value=Hall_Parameter.shift
  If Action Subsystem1 : Subsystem  TreatAsAtomicUnit=on
  If Action Subsystem2 : Subsystem  TreatAsAtomicUnit=on
  If Action Subsystem3 : Subsystem  TreatAsAtomicUnit=on
  If1 : If  IfExpression=u1 > 6.283185307  ElseIfExpressions=u1<0
  Merge1 : Merge  Inputs=3
  Subtract1 : Sum
  Angle_output : Outport
  wires:
  Angle_input/1 -> Subtract1/1
  Angle_offset/1 -> Subtract1/2  "Control_ModeCommand"
  If1/1 -> If Action Subsystem2/Action
  If1/3 -> If Action Subsystem1/Action
  If Action Subsystem2/1(Out1) -> Merge1/1
  Subtract1/1 -> If Action Subsystem3/1(In1), If Action Subsystem1/1(In1), If Action Subsystem2/1(In1), If1/1
  If Action Subsystem1/1(Out1) -> Merge1/3
  If Action Subsystem3/1(Out1) -> Merge1/2
  If1/2 -> If Action Subsystem3/Action
  Merge1/1 -> Angle_output/1

== system PMSM_FOC_Traction/Motor_Control/Motor_Control_Funtion/Angle_Speed_100us/SpeedAndAngle/Subsystem/Subsystem ==
  Action Port : ActionPort  ActionPortLabel=if(u1 ==1)
  Commutation : Subsystem
  Duty : Constant  Value=Hall_Parameter.Start_duty*4200  SampleTime=-1
  Gate : Outport  VectorParamsAs1DForOutWhenUnconnected=off
  Duty_Set : Outport  Port=2  VectorParamsAs1DForOutWhenUnconnected=off
  wires:
  Duty/1 -> Duty_Set/1
  Commutation/1(S) -> Gate/1

== system PMSM_FOC_Traction/Motor_Control/Motor_Control_Funtion/Angle_Speed_100us/SpeedAndAngle/Subsystem/Subsystem1 ==
  Hall : Inport
  Action Port : ActionPort  ActionPortLabel=elseif(u1 ==2)
  Commutation : Subsystem
  Duty : Constant  Value=Hall_Parameter.Start_duty*4200  SampleTime=-1
  Gate : Outport  VectorParamsAs1DForOutWhenUnconnected=off
  Duty_Set : Outport  Port=2  VectorParamsAs1DForOutWhenUnconnected=off
  wires:
  Duty/1 -> Duty_Set/1
  Hall/1 -> Commutation/1(Hall)
  Commutation/1(S) -> Gate/1

== system PMSM_FOC_Traction/Motor_Control/Motor_Control_Funtion/Angle_Speed_100us/SpeedAndAngle/Subsystem1/Subsystem ==
  In1 : Inport
  In2 : Inport  Port=2
  Action Port : ActionPort  ActionPortLabel=if(u1 ==1 | u1 ==2)
  Out1 : Outport
  Out2 : Outport  Port=2
  wires:
  In1/1 -> Out1/1
  In2/1 -> Out2/1

== system PMSM_FOC_Traction/Motor_Control/Motor_Control_Funtion/Angle_Speed_100us/SpeedAndAngle/Subsystem1/Subsystem1 ==
  In1 : Inport
  In2 : Inport  Port=2
  Action Port : ActionPort  ActionPortLabel=elseif(u1==3)
  Out1 : Outport
  Out2 : Outport  Port=2
  wires:
  In1/1 -> Out1/1
  In2/1 -> Out2/1
